simulink model "run_quadrotor_2020a_working"  (R2020a)
settings: Solver=ode45  StartTime=0.0  StopTime=10000  RelTol=1e-3  EnableMultiTasking=on
InitFcn:
  | addpath('display/')
  | addpath('parameters/')
  | addpath('quadrotor_model')
  | addpath('tools/')
  | addpath('libs/RealTima_Pacer')
  | aerosonde_parameters
  | simulation_parameters
undefined symbols (not defined in the file or in its folder): drawQuadrotor, plotmavstatevariables, SAMPLE_TIME
libraries: simulink x14, realtime_pacer_lib x1
settings Model: Creator=beard  LastModifiedBy=andrey
settings DataIOCC: LimitDataPoints=on  SaveFormat=Array  SignalLoggingSaveFormat=ModelDataLogs  ReturnWorkspaceOutputs=off
settings OptimizationCC: ExpressionDepthLimit=2147483647  InitFltsAndDblsToZero=on  LifeSpan=inf
settings DebuggingCC: UnderspecifiedInitializationDetection=Classic  MergeDetectMultiDrivingBlocksExec=none  SolverPrmCheckMsg=warning  FcnCallInpInsideContextMsg=warning  AllowSymbolicDim=off  StateNameClashWarn=warning  SFUnexpectedBacktrackingDiag=warning  SFNoUnconditionalDefaultTransitionDiag=warning  SFExecutionAtInitializationDiag=none  ArithmeticOperatorsInVariantConditions=warning
settings HardwareCC: ProdBitPerPointer=32  ProdBitPerSizeT=32  ProdBitPerPtrDiffT=32  ProdLargestAtomicFloat=None  ProdIntDivRoundTo=Undefined  ProdEndianess=Unspecified  ProdWordSize=32  ProdHWDeviceType=32-bit Generic
settings ModelReferenceCC: PropagateSignalLabelsOutOfModel=off
settings SFSimCC: SimUseLocalCustomCode=off  CustomCodeUndefinedFunction=UseInterfaceOnly
settings RTWCC: RTWUseLocalCustomCode=off
settings CodeAppCC: StateflowObjectComments=on
settings GRTTargetCC: TargetLangStandard=C89/C90 (ANSI)  CombineOutputUpdateFcns=off  GRTInterface=on
settings ConfigComp: CovMetricSettings=dw  CovSaveCumulativeToWorkspaceVar=on  CovSaveSingleToWorkspaceVar=on  CovExternalEMLEnable=off  CovSFcnEnable=off

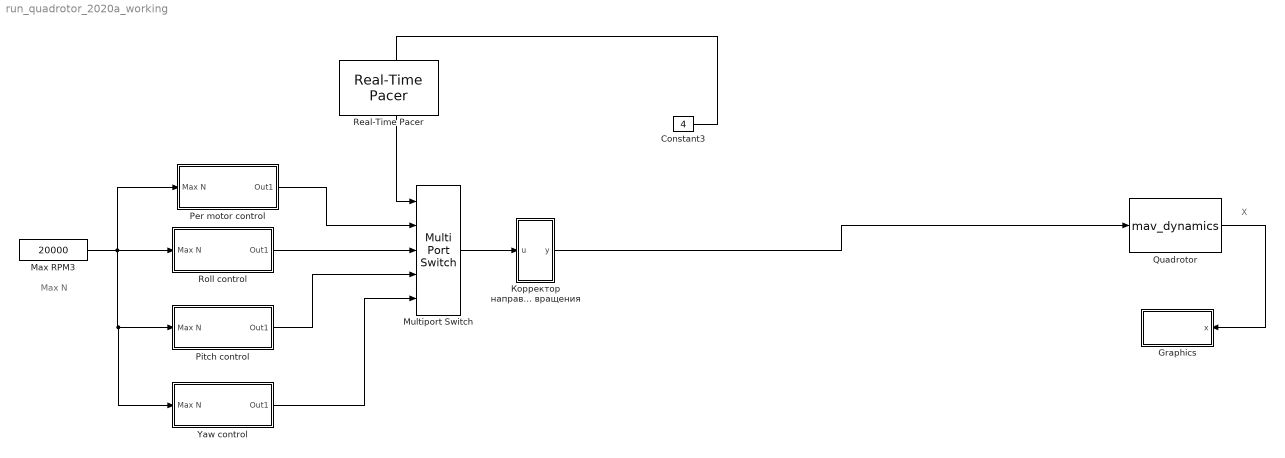
== system run_quadrotor_2020a_working ==
  note: X
  note: Max N
  Constant3 : Constant  Value=4
  Graphics : Subsystem
      mask Display: image(imread('../chap2/tv.jpg'))
  Max RPM3 : Constant  Value=20000  SampleTime=SAMPLE_TIME
  Multiport Switch : MultiPortSwitch  Inputs=4
  Per motor control : Subsystem
  Pitch control : Subsystem
  Quadrotor : S-Function  FunctionName=mav_dynamics  Parameters=MAV  SFunctionDeploymentMode=off  EnableBusSupport=off
  Real-Time Pacer : realtime_pacer_lib/Real-Time Pacer  simTimePerRealTime=1
  Roll control : Subsystem
  Yaw control : Subsystem
  Корректор направлений вращения : MATLAB Function  TreatAsAtomicUnit=on
  wires:
  Quadrotor/1 -> Graphics/1(x)
  Max RPM3/1 -> Roll control/1(Max N), Yaw control/1(Max N), Pitch control/1(Max N), Per motor control/1(Max N)
  Constant3/1 -> Multiport Switch/1
  Multiport Switch/1 -> Корректор направлений вращения/1(u)
  Per motor control/1(Out1) -> Multiport Switch/2
  Roll control/1(Out1) -> Multiport Switch/3
  Pitch control/1(Out1) -> Multiport Switch/4
  Yaw control/1(Out1) -> Multiport Switch/5
  Корректор направлений вращения/1(y) -> Quadrotor/1

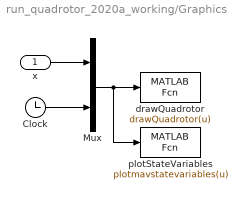
== system run_quadrotor_2020a_working/Graphics ==
  x : Inport
  Clock : Clock
  Mux : Mux  Inputs=2
  drawQuadrotor : MATLABFcn  MATLABFcn=drawQuadrotor(u)  OutputDimensions=0  SampleTime=0.1
  plotStateVariables : MATLABFcn  MATLABFcn=plotmavstatevariables(u)  OutputDimensions=0
  wires:
  x/1 -> Mux/1
  Clock/1 -> Mux/2
  Mux/1 -> plotStateVariables/1, drawQuadrotor/1

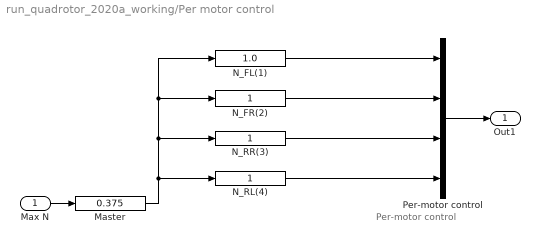
== system run_quadrotor_2020a_working/Per motor control ==
  note: Per-motor control
  Max N : Inport
  Master : simulink/Math Operations/Slider Gain  gain=0.375  low=0  high=1
  N_FL(1) : simulink/Math Operations/Slider Gain  gain=1.0  low=0  high=1
  N_FR(2) : simulink/Math Operations/Slider Gain  gain=1  low=0  high=1
  N_RL(4) : simulink/Math Operations/Slider Gain  gain=1  low=0  high=1
  N_RR(3) : simulink/Math Operations/Slider Gain  gain=1  low=0  high=1
  Per-motor control : Mux
  Out1 : Outport
  wires:
  N_RL(4)/1 -> Per-motor control/4
  N_FL(1)/1 -> Per-motor control/1
  N_FR(2)/1 -> Per-motor control/2
  Per-motor control/1 -> Out1/1
  Master/1 -> N_RL(4)/1, N_RR(3)/1, N_FR(2)/1, N_FL(1)/1
  N_RR(3)/1 -> Per-motor control/3
  Max N/1 -> Master/1

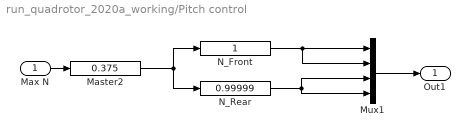
== system run_quadrotor_2020a_working/Pitch control ==
  Max N : Inport
  Master2 : simulink/Math Operations/Slider Gain  gain=0.375  low=0  high=1
  Mux1 : Mux
  N_Front : simulink/Math Operations/Slider Gain  gain=1  low=0  high=1
  N_Rear : simulink/Math Operations/Slider Gain  gain=0.99999  low=0  high=1
  Out1 : Outport
  wires:
  N_Rear/1 -> Mux1/3, Mux1/4
  Master2/1 -> N_Rear/1, N_Front/1
  N_Front/1 -> Mux1/2, Mux1/1
  Max N/1 -> Master2/1
  Mux1/1 -> Out1/1

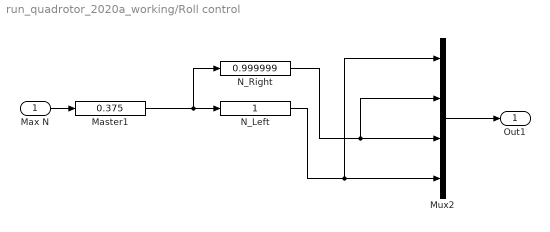
== system run_quadrotor_2020a_working/Roll control ==
  Max N : Inport
  Master1 : simulink/Math Operations/Slider Gain  gain=0.375  low=0  high=1
  Mux2 : Mux
  N_Left : simulink/Math Operations/Slider Gain  gain=1  low=0  high=1
  N_Right : simulink/Math Operations/Slider Gain  gain=0.999999  low=0  high=1
  Out1 : Outport
  wires:
  N_Right/1 -> Mux2/2, Mux2/3
  Master1/1 -> N_Left/1, N_Right/1
  N_Left/1 -> Mux2/1, Mux2/4
  Max N/1 -> Master1/1
  Mux2/1 -> Out1/1

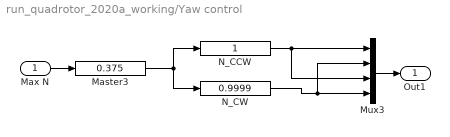
== system run_quadrotor_2020a_working/Yaw control ==
  Max N : Inport
  Master3 : simulink/Math Operations/Slider Gain  gain=0.375  low=0  high=1
  Mux3 : Mux
  N_CCW : simulink/Math Operations/Slider Gain  gain=1  low=0  high=1
  N_CW : simulink/Math Operations/Slider Gain  gain=0.9999  low=0  high=1
  Out1 : Outport
  wires:
  N_CCW/1 -> Mux3/3, Mux3/1
  Master3/1 -> N_CW/1, N_CCW/1
  N_CW/1 -> Mux3/2, Mux3/4
  Max N/1 -> Master3/1
  Mux3/1 -> Out1/1

== matlab function run_quadrotor_2020a_working/Корректор направлений вращения ==
  data: u input; y output
function y = fcn(u)

    y = [1 -1 1 -1]' .* u;
